simulink model "DiscreteDroneModelV2"  (R2024a)
settings: Solver=VariableStepAuto  StartTime=0.0  StopTime=20  RelTol=1e-3
PreLoadFcn:
  | run("StateSpace.m")
  | run("QuadcopterAttributes.m")
  | run("Motormixing.m")
  | run("reduced_state_space.m")
  | run("LQI_reduced.m")
values from neighbouring files (symbols this model uses):
  A_r = [0 0 0 0 1 0 0 0 ... (first row only)    [reduced_state_space.m]
  B = [0 0 0 0 ... (first row only)    [StateSpace.m]
  B_r = [0 0 0 0 ... (first row only)    [reduced_state_space.m]
  C = [1 0 0 0 0 0 0 0 0 0 0 0 ... (first row only)    [StateSpace.m]
  C_r = ctrb(A,B)    [OptimalControlLQCalculations.m]    (also in reduced_state_space.m = [1 0 0 0 0 0 0 0)
  dis = 81.17 * 10^-3    (= 0.08117)    [Motormixing.m]
  drag_co = torque_Nm / no_rot^2    (= 9.75332775919e-12)    [QuadcopterAttributes.m]
  E = [1 0 0 0 0 0 0 0;]    [LQI_reduced.m]
  g = 9.81    [StateSpace.m]
  K_LQR_reduced = lqr(A_r, B_r, Q_reduced, R_reduced, 0)    [LQR_reduced.m]    (also in reduced_state_space.m)
  K_mm = inv(K_mm_FtoU)    [Motormixing.m]
  Ki_lqi = K_lqi(:,13:16)    [LQI.m]    (also in LQICalculations.m)
  Ki_lqi_reduced = K_lqi_reduced(:,9)    [LQI_reduced.m]
  KV_rating = 2800    [QuadcopterAttributes.m]
  Kx_lqi = K_lqi(:,1:12)    [LQI.m]    (also in LQICalculations.m)
  Kx_lqi_reduced = K_lqi_reduced(:,1:8)    [LQI_reduced.m]
  lift_co = thrust_N / no_rot^2    (= 5.88883004597e-10)    [QuadcopterAttributes.m]
  m = 0.5    [StateSpace.m]
  r = 0.25    [StateSpace.m]
  x0_r = [0;0;0;0;0;0;0;0;]    [reduced_state_space.m]
undefined symbols (not defined in the file or in its folder): A, battery_voltage, C_lqi, I_p, sigma
libraries: sim3dlib x2, uavsim3dlib x2, shared6dof x1
settings Model: Creator=Henrik  LastModifiedBy=felih

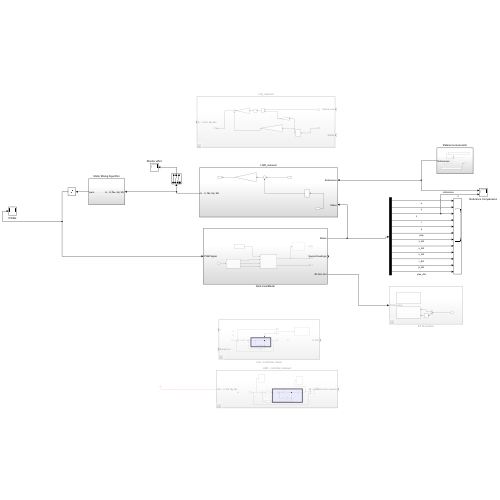
[thumbnail: Simulink's stored preview of the top-level diagram]
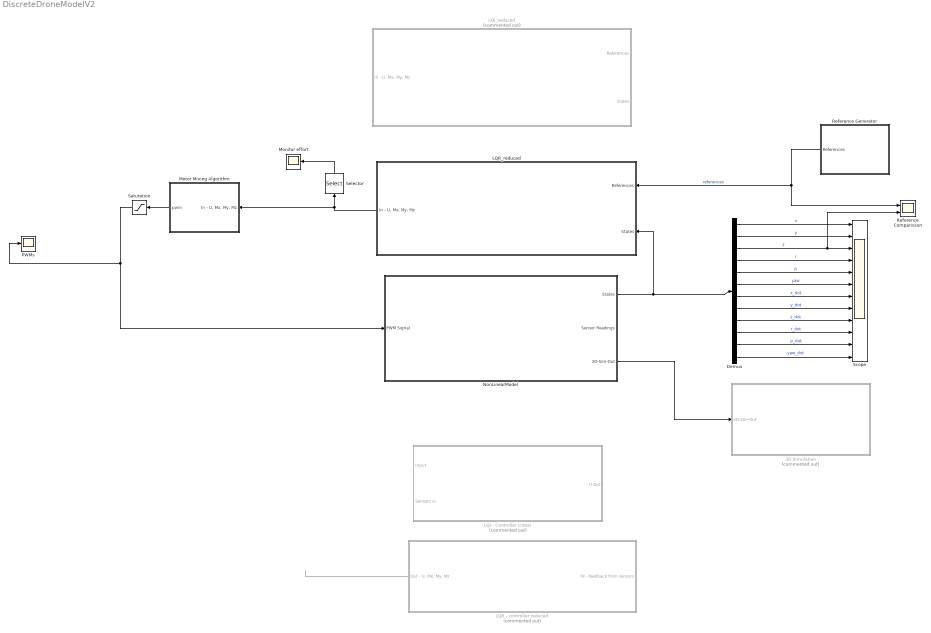
== system DiscreteDroneModelV2 ==
  3D Simulation : Subsystem  Commented=on
  Demux : Demux  Outputs=12
  LQI - Controller Linear : Subsystem  Commented=on
  LQI_reduced : Subsystem  Commented=on
  LQR - controller reduced : Subsystem  Commented=on
  LQR_reduced : Subsystem
  Monitor effort : Scope
  Motor Mixing Algorithm : Subsystem
  NonLinearModel : Subsystem
  PWMs : Scope
  Reference Comparisson : Scope  NumInputPorts=2
  Reference Generator : Subsystem
  Saturation : Saturate  UpperLimit=255  LowerLimit=0
  Scope : Scope  NumInputPorts=12
  Selector : Selector  InputPortWidth=4  IndexOptions=Index vector (dialog)  Indices=[1 2 3]  OutputSizes=1
  wires:
  LQR - controller reduced/1("Out - U, Mx, My, Mz") -> ?
  Demux/1 -> Scope/1  "x"
  Demux/2 -> Scope/2  "y"
  Demux/3 -> Reference Comparisson/2, Scope/3  "z"
  Demux/4 -> Scope/4  "r"
  Demux/5 -> Scope/5  "p"
  Demux/6 -> Scope/6  "yaw"
  Demux/7 -> Scope/7  "x_dot"
  Demux/8 -> Scope/8  "y_dot"
  Demux/9 -> Scope/9  "z_dot"
  Demux/10 -> Scope/10  "r_dot"
  Demux/11 -> Scope/11  "p_dot"
  Demux/12 -> Scope/12  "yaw_dot"
  NonLinearModel/1(States) -> LQR_reduced/2(States), Demux/1
  Motor Mixing Algorithm/1(pwm) -> Saturation/1
  Saturation/1 -> PWMs/1, NonLinearModel/1(PWM Signal)
  LQR_reduced/1("In - U, Mx, My, Mz") -> Selector/1, Motor Mixing Algorithm/1("In - U, Mx, My, Mz")
  Reference Generator/1(References) -> Reference Comparisson/1, LQR_reduced/1(References)  "references"
  Selector/1 -> Monitor effort/1
  NonLinearModel/3(3D-Sim-Out) -> 3D Simulation/1(3D-Sim-Out)

== system DiscreteDroneModelV2/3D Simulation ==
  3D-Sim-Out : Inport
  Demux : Demux  Outputs=2
  Flip : DSPFlip
  Simulation 3D Scene Configuration : sim3dlib/Simulation 3D Scene Configuration  Priority=0  ProjectFormat=Default Scenes  SceneDesc=US city block  ProjectName=C:\Program Files\MATLAB\R2024a\toolbox\shared\sim3d_projects\automotive_project_windows\UE\WindowsNoEditor\VehicleSimulation.exe  ScenePath=/Game/Maps/USCityBlock  EnableOpenDRIVE=off  vehTagList={'Scene Origin';'SimulinkVehicle1'}  vehTag=SimulinkVehicle1  FreeCameraInitialTranslation=[0, 0, 0]  FreeCameraDefaultInitialTranslation=[-6, 0, 2]  FreeCameraInitialRotation=[0, 0, 0]  FreeCameraDefaultInitialRotation=[0, -15, 0]  OpVisEn=off  Ts=1/60  EnableWindow=on  EnableRemoteAccess=off  EnableWeather=off  SunAzimuth=90  SunAltitude=40.0  EnableGeospatialSun=off  Latitude=0  Longitude=0  Date=2023-01-01  Time=10:30:00  GeoTimeZone=-5.0  SunDaylightSaving=off  wind=1  clouds=10  EnableVolumetricClouds=off  CloudCoverage=0  CloudAltitude=6  fog=30.0  rain=0  RaindropsEffect=off  SnowDensity=0  EnableGeospatial=off  UseTrueOrigin=off  OriginHeight=200  OriginLatitude=40.744652  OriginLongitude=-73.988864  MapStyle=Aerial  AdditionalAssetIDs=[]  UseAdvancedSunSky=off  SolarTime=11  TimeZone=-5  Day=21  Month=9  Year=2022  UseDaylightSavingTime=on  DSTStartDay=10  DSTStartMonth=3  DSTEndDay=3  DSTEndMonth=11  DSTSwitchHour=2  sensorTag=MainCamera1  sensorId=1  sensorName=MainCamera1  mountLoc=Origin  offsetFlag=off  tmountOffset=[0, 0, 0]  rmountOffset=[0, 0, 0]  HorizontalResolution=1280  VerticalResolution=720  HorizontalFOV=60  mountPoint=[0 0 0]  mountOrientation=[0 0 0]  aMode=4  ID=1  GeoTrigger=Inactive
      settings: LibrarySourceBlock=uavsim3dlib/Simulation 3D Scene Configuration
  Simulation 3D UAV Vehicle : uavsim3dlib/Simulation 3D UAV Vehicle  Priority=-1  Mesh=Quadrotor  MeshPath=/MathWorksUAVContent/UAVs/HexaRotorUAV/HexaRotor.HexaRotor  Color=Silver  ActorName=SimulinkVehicle1  UseGlobalFrame=off  InitialTranslation=[0 0 0]  InitialRotation=[0 0 0]  InitialTranslationGlobal=[0 0 0]  InitialGeoOrigin=[0 0 0]  InitialRotationGlobal=[0 0 0]  SampleTime=-1  ActorType=SimulinkVehicle  ID=1  aMode=4  ActorTag=SimulinkVehicle1
  wires:
  Demux/1 -> Simulation 3D UAV Vehicle/1
  Flip/1 -> Simulation 3D UAV Vehicle/2
  Demux/2 -> Flip/1
  3D-Sim-Out/1 -> Demux/1

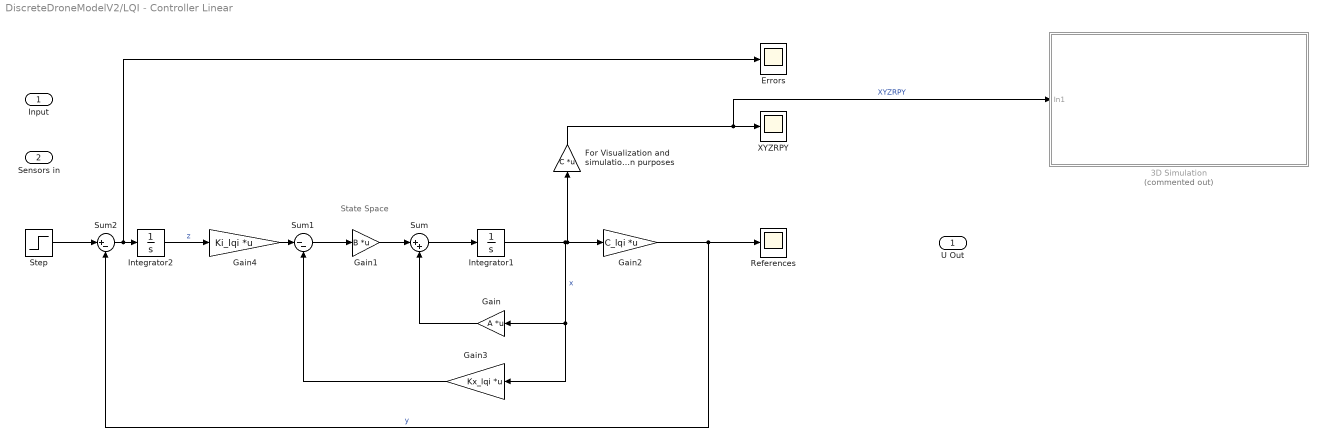
== system DiscreteDroneModelV2/LQI - Controller Linear ==
  note: State Space
  Input : Inport
  Sensors in : Inport  Port=2
  3D Simulation : Subsystem  Commented=on
  Errors : Scope
  For Visualization and simulation purposes : Gain  Gain=C  Multiplication=Matrix(K*u)
  Gain : Gain  Gain=A  Multiplication=Matrix(K*u)
  Gain1 : Gain  Gain=B  Multiplication=Matrix(K*u)
  Gain2 : Gain  Gain=C_lqi  Multiplication=Matrix(K*u)
  Gain3 : Gain  Gain=Kx_lqi  Multiplication=Matrix(K*u)
  Gain4 : Gain  Gain=Ki_lqi  Multiplication=Matrix(K*u)
  Integrator1 : Integrator
  Integrator2 : Integrator
  References : Scope
  Step : Step  Before=[0;0;0;0]  After=[20;-3;100;3]  SampleTime=0
  Sum : Sum  Inputs=|++
  Sum1 : Sum  Inputs=|--
  Sum2 : Sum  Inputs=|+-
  XYZRPY : Scope
  U Out : Outport
  wires:
  Gain/1 -> Sum/2
  Gain1/1 -> Sum/1
  Sum/1 -> Integrator1/1
  Integrator1/1 -> For Visualization and simulation purposes/1, Gain2/1, Gain3/1, Gain/1  "x"
  Gain2/1 -> References/1, Sum2/2  "y"
  Sum1/1 -> Gain1/1
  Gain3/1 -> Sum1/2
  Step/1 -> Sum2/1
  Sum2/1 -> Errors/1, Integrator2/1
  Integrator2/1 -> Gain4/1  "z"
  Gain4/1 -> Sum1/1
  For Visualization and simulation purposes/1 -> 3D Simulation/1(In1), XYZRPY/1  "XYZRPY"

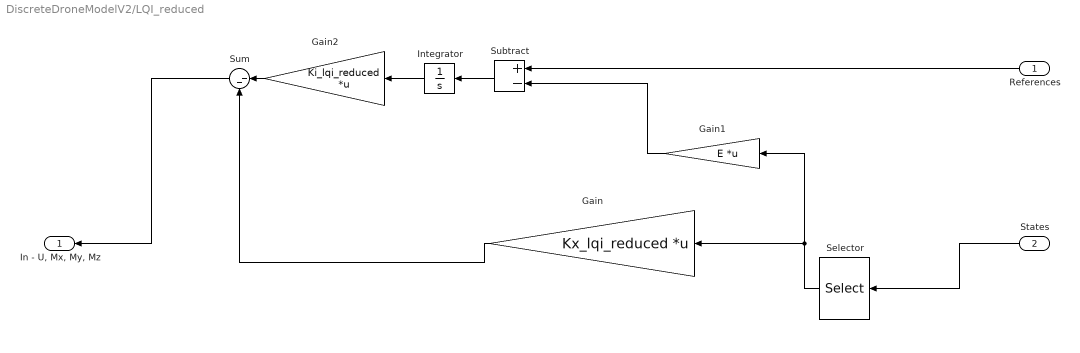
== system DiscreteDroneModelV2/LQI_reduced ==
  References : Inport
  States : Inport  Port=2
  Gain : Gain  Gain=Kx_lqi_reduced  Multiplication=Matrix(K*u)
  Gain1 : Gain  Gain=E  Multiplication=Matrix(K*u)
  Gain2 : Gain  Gain=Ki_lqi_reduced  Multiplication=Matrix(K*u)
  Integrator : Integrator
  Selector : Selector  InputPortWidth=12  IndexOptions=Index vector (dialog)  Indices=[3 4 5 6 9 10 11 12]  OutputSizes=1
  Subtract : Sum  Inputs=+-
  Sum : Sum  Inputs=|--
  "In - U, Mx, My, Mz" : Outport
  wires:
  Selector/1 -> Gain1/1, Gain/1
  Subtract/1 -> Integrator/1
  Gain1/1 -> Subtract/2
  Sum/1 -> "In - U, Mx, My, Mz"/1
  Gain/1 -> Sum/2
  Gain2/1 -> Sum/1
  Integrator/1 -> Gain2/1
  References/1 -> Subtract/1
  States/1 -> Selector/1

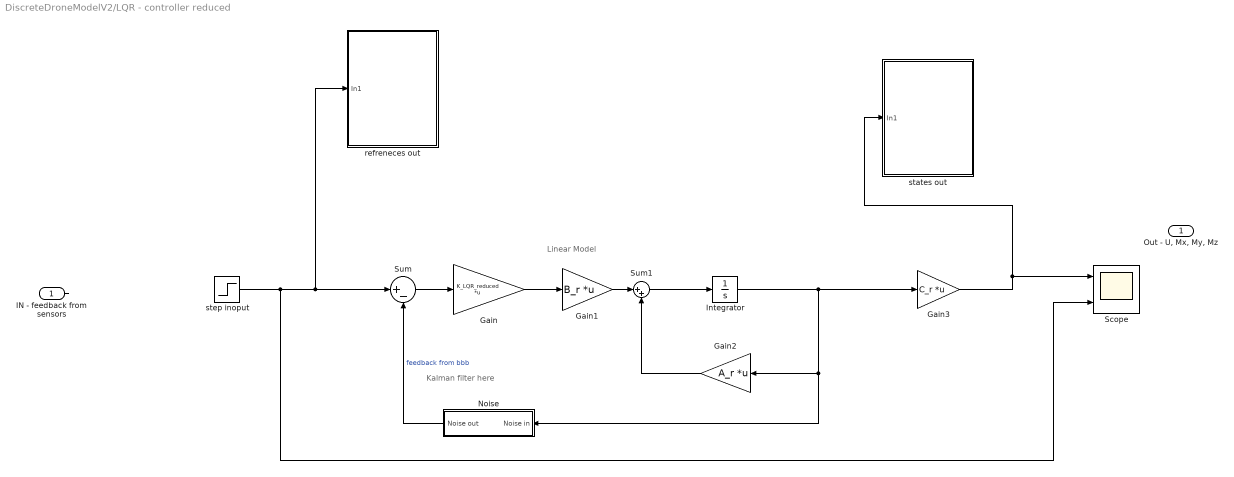
== system DiscreteDroneModelV2/LQR - controller reduced ==
  note: Linear Model
  note: Kalman filter here
  IN - feedback from sensors : Inport
  Gain : Gain  Gain=K_LQR_reduced  Multiplication=Matrix(K*u)
  Gain1 : Gain  Gain=B_r  Multiplication=Matrix(K*u)
  Gain2 : Gain  Gain=A_r  Multiplication=Matrix(K*u)
  Gain3 : Gain  Gain=C_r  Multiplication=Matrix(K*u)
  Integrator : Integrator  InitialCondition=x0_r
  Noise : Subsystem
  Scope : Scope  NumInputPorts=2
  Sum : Sum  Inputs=|+-
  Sum1 : Sum  Inputs=|++
  refreneces out : Subsystem
  states out : Subsystem
  step inoput : Step  Time=0  Before=zeros(8,1)  After=[0;1;0;0;0;0;0;0]  SampleTime=0
  "Out - U, Mx, My, Mz" : Outport
  wires:
  IN - feedback from sensors/1 -> ?
  Sum/1 -> Gain/1
  Gain/1 -> Gain1/1
  Gain1/1 -> Sum1/1
  Gain2/1 -> Sum1/2
  Sum1/1 -> Integrator/1
  Integrator/1 -> Gain2/1, Noise/1(Noise in), Gain3/1
  Gain3/1 -> states out/1(In1), Scope/1
  step inoput/1 -> Scope/2, refreneces out/1(In1), Sum/1
  Noise/1(Noise out) -> Sum/2  "feedback from bbb"

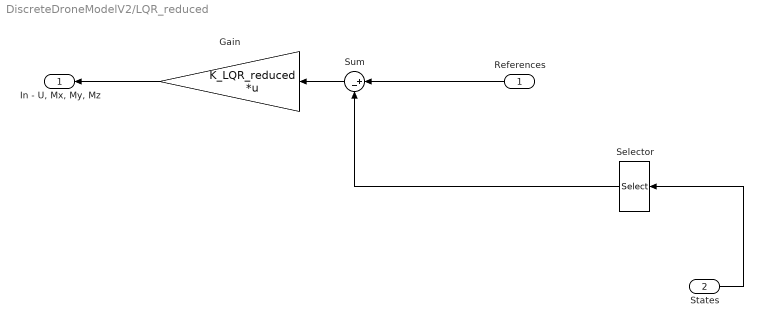
== system DiscreteDroneModelV2/LQR_reduced ==
  References : Inport
  States : Inport  Port=2
  Gain : Gain  Gain=K_LQR_reduced  Multiplication=Matrix(K*u)
  Selector : Selector  InputPortWidth=12  IndexOptions=Index vector (dialog)  Indices=[3 4 5 6 9 10 11 12]  OutputSizes=1
  Sum : Sum  Inputs=|+-
  "In - U, Mx, My, Mz" : Outport
  wires:
  Gain/1 -> "In - U, Mx, My, Mz"/1
  Selector/1 -> Sum/2
  Sum/1 -> Gain/1
  States/1 -> Selector/1
  References/1 -> Sum/1

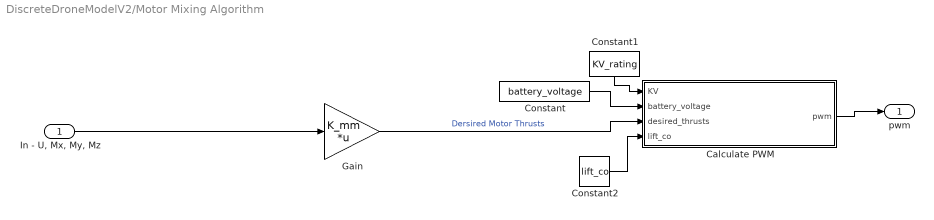
== system DiscreteDroneModelV2/Motor Mixing Algorithm ==
  "In - U, Mx, My, Mz" : Inport
  Calculate PWM : MATLAB Function  TreatAsAtomicUnit=on
  Constant : Constant  Value=battery_voltage
  Constant1 : Constant  Value=KV_rating
  Constant2 : Constant  Value=lift_co
  Gain : Gain  Gain=K_mm  Multiplication=Matrix(K*u)
  pwm : Outport
  wires:
  "In - U, Mx, My, Mz"/1 -> Gain/1
  Gain/1 -> Calculate PWM/3(desired_thrusts)  "Dersired Motor Thrusts"
  Constant/1 -> Calculate PWM/2(battery_voltage)
  Constant1/1 -> Calculate PWM/1(KV)
  Calculate PWM/1(pwm) -> pwm/1
  Constant2/1 -> Calculate PWM/4(lift_co)

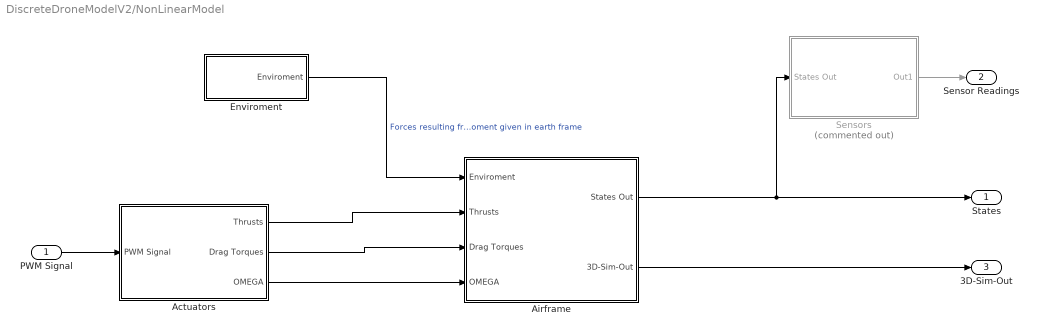
== system DiscreteDroneModelV2/NonLinearModel ==
  PWM Signal : Inport
  Actuators : Subsystem
  Airframe : Subsystem
  Enviroment : Subsystem
  Sensors : Subsystem  Commented=on
  States : Outport
  Sensor Readings : Outport  Port=2
  3D-Sim-Out : Outport  Port=3
  wires:
  PWM Signal/1 -> Actuators/1(PWM Signal)
  Airframe/1(States Out) -> Sensors/1(States Out), States/1
  Enviroment/1(Enviroment) -> Airframe/1(Enviroment)  "Forces resulting from enviroment given in earth frame"
  Actuators/1(Thrusts) -> Airframe/2(Thrusts)
  Airframe/2(3D-Sim-Out) -> 3D-Sim-Out/1
  Actuators/2(Drag Torques) -> Airframe/3(Drag Torques)
  Actuators/3(OMEGA) -> Airframe/4(OMEGA)
  Sensors/1(Out1) -> Sensor Readings/1

== system DiscreteDroneModelV2/Reference Generator ==
  Constant : Constant  Value=[0;0;0;0;0;0;0]
  Constant1 : Constant  Value=[0.35;0;0;0;0;0;0;0]
  Mux : Mux  Inputs=2
  Step : Step  Time=0  After=0.35  SampleTime=0
  References : Outport
  wires:
  Step/1 -> ?
  Constant/1 -> Mux/2
  Mux/1 -> ?
  Constant1/1 -> References/1

== system DiscreteDroneModelV2/LQI - Controller Linear/3D Simulation ==
  In1 : Inport
  Demux : Demux  Outputs=2
  Flip : DSPFlip
  Simulation 3D Scene Configuration : sim3dlib/Simulation 3D Scene Configuration  Priority=0  ProjectFormat=Default Scenes  SceneDesc=US city block  ProjectName=C:\Program Files\MATLAB\R2024a\toolbox\shared\sim3d_projects\automotive_project_windows\UE\WindowsNoEditor\VehicleSimulation.exe  ScenePath=/Game/Maps/USCityBlock  EnableOpenDRIVE=off  vehTagList={'Scene Origin';'SimulinkVehicle1'}  vehTag=SimulinkVehicle1  FreeCameraInitialTranslation=[0, 0, 0]  FreeCameraDefaultInitialTranslation=[-6, 0, 2]  FreeCameraInitialRotation=[0, 0, 0]  FreeCameraDefaultInitialRotation=[0, -15, 0]  OpVisEn=off  Ts=1/60  EnableWindow=on  EnableRemoteAccess=off  EnableWeather=off  SunAzimuth=90  SunAltitude=40.0  EnableGeospatialSun=off  Latitude=0  Longitude=0  Date=2023-01-01  Time=10:30:00  GeoTimeZone=-5.0  SunDaylightSaving=off  wind=1  clouds=10  EnableVolumetricClouds=off  CloudCoverage=0  CloudAltitude=6  fog=30.0  rain=0  RaindropsEffect=off  SnowDensity=0  EnableGeospatial=off  UseTrueOrigin=off  OriginHeight=200  OriginLatitude=40.744652  OriginLongitude=-73.988864  MapStyle=Aerial  AdditionalAssetIDs=[]  UseAdvancedSunSky=off  SolarTime=11  TimeZone=-5  Day=21  Month=9  Year=2022  UseDaylightSavingTime=on  DSTStartDay=10  DSTStartMonth=3  DSTEndDay=3  DSTEndMonth=11  DSTSwitchHour=2  sensorTag=MainCamera1  sensorId=1  sensorName=MainCamera1  mountLoc=Origin  offsetFlag=off  tmountOffset=[0, 0, 0]  rmountOffset=[0, 0, 0]  HorizontalResolution=1280  VerticalResolution=720  HorizontalFOV=60  mountPoint=[0 0 0]  mountOrientation=[0 0 0]  aMode=4  ID=1  GeoTrigger=Inactive
      settings: LibrarySourceBlock=uavsim3dlib/Simulation 3D Scene Configuration
  Simulation 3D UAV Vehicle : uavsim3dlib/Simulation 3D UAV Vehicle  Priority=-1  Mesh=Quadrotor  MeshPath=/MathWorksUAVContent/UAVs/HexaRotorUAV/HexaRotor.HexaRotor  Color=Silver  ActorName=SimulinkVehicle1  UseGlobalFrame=off  InitialTranslation=[0 0 0]  InitialRotation=[0 0 0]  InitialTranslationGlobal=[0 0 0]  InitialGeoOrigin=[0 0 0]  InitialRotationGlobal=[0 0 0]  SampleTime=-1  ActorType=SimulinkVehicle  ID=1  aMode=4  ActorTag=SimulinkVehicle1
  wires:
  Demux/1 -> Simulation 3D UAV Vehicle/1
  Flip/1 -> Simulation 3D UAV Vehicle/2
  Demux/2 -> Flip/1
  In1/1 -> Demux/1

== system DiscreteDroneModelV2/LQR - controller reduced/Noise ==
  Noise in : Inport
  Random Number12 : RandomNumber  Mean=0.1  Variance=0.1  SampleTime=0.001
  Sum2 : Sum  Inputs=|++
  Transfer Fcn12 : TransferFcn  Numerator=[50 0]  Denominator=[50 1]
  X noise1 : Gain  Gain=[0;1;0;0;0;0;0;0]  Multiplication=Matrix(K*u)
  Noise out : Outport
  wires:
  X noise1/1 -> Sum2/2
  Transfer Fcn12/1 -> X noise1/1
  Random Number12/1 -> Transfer Fcn12/1
  Noise in/1 -> Sum2/1
  Sum2/1 -> Noise out/1

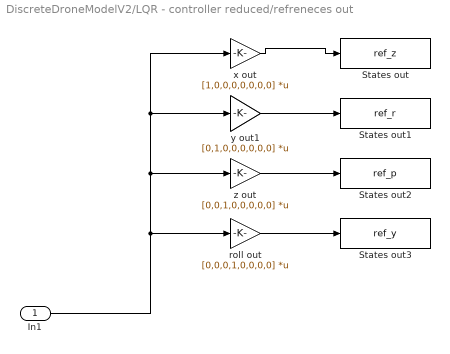
== system DiscreteDroneModelV2/LQR - controller reduced/refreneces out ==
  In1 : Inport
  States out : ToWorkspace  VariableName=ref_z  SaveFormat=Timeseries  SampleTime=-1
  States out1 : ToWorkspace  VariableName=ref_r  SaveFormat=Timeseries  SampleTime=-1
  States out2 : ToWorkspace  VariableName=ref_p  SaveFormat=Timeseries  SampleTime=-1
  States out3 : ToWorkspace  VariableName=ref_y  SaveFormat=Timeseries  SampleTime=-1
  roll out : Gain  Gain=[0,0,0,1,0,0,0,0]  Multiplication=Matrix(K*u)
  x out : Gain  Gain=[1,0,0,0,0,0,0,0]  Multiplication=Matrix(K*u)
  y out1 : Gain  Gain=[0,1,0,0,0,0,0,0]  Multiplication=Matrix(K*u)
  z out : Gain  Gain=[0,0,1,0,0,0,0,0]  Multiplication=Matrix(K*u)
  wires:
  z out/1 -> States out2/1
  In1/1 -> roll out/1, z out/1, y out1/1, x out/1
  y out1/1 -> States out1/1
  x out/1 -> States out/1
  roll out/1 -> States out3/1

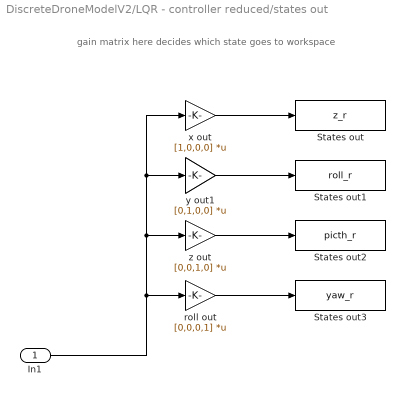
== system DiscreteDroneModelV2/LQR - controller reduced/states out ==
  note: gain matrix here decides which state goes to workspace
  In1 : Inport
  States out : ToWorkspace  VariableName=z_r  SaveFormat=Timeseries  SampleTime=-1
  States out1 : ToWorkspace  VariableName=roll_r  SaveFormat=Timeseries  SampleTime=-1
  States out2 : ToWorkspace  VariableName=picth_r  SaveFormat=Timeseries  SampleTime=-1
  States out3 : ToWorkspace  VariableName=yaw_r  SaveFormat=Timeseries  SampleTime=-1
  roll out : Gain  Gain=[0,0,0,1]  Multiplication=Matrix(K*u)
  x out : Gain  Gain=[1,0,0,0]  Multiplication=Matrix(K*u)
  y out1 : Gain  Gain=[0,1,0,0]  Multiplication=Matrix(K*u)
  z out : Gain  Gain=[0,0,1,0]  Multiplication=Matrix(K*u)
  wires:
  y out1/1 -> States out1/1
  In1/1 -> x out/1, y out1/1, z out/1, roll out/1
  roll out/1 -> States out3/1
  z out/1 -> States out2/1
  x out/1 -> States out/1

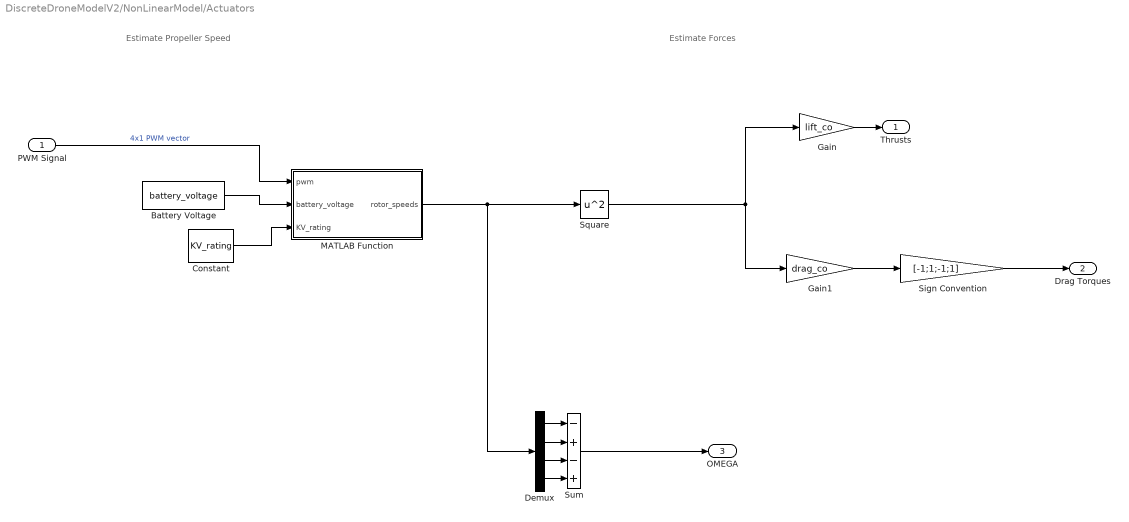
== system DiscreteDroneModelV2/NonLinearModel/Actuators ==
  note: Estimate Forces
  note: Estimate Propeller Speed
  PWM Signal : Inport
  Battery Voltage : Constant  Value=battery_voltage
  Constant : Constant  Value=KV_rating
  Demux : Demux
  Gain : Gain  Gain=lift_co
  Gain1 : Gain  Gain=drag_co
  MATLAB Function : MATLAB Function  TreatAsAtomicUnit=on
  Sign Convention : Gain  Gain=[-1;1;-1;1]
  Square : Math  Operator=square
  Sum : Sum  Inputs=-+-+
  Thrusts : Outport
  Drag Torques : Outport  Port=2
  OMEGA : Outport  Port=3
  wires:
  Constant/1 -> MATLAB Function/3(KV_rating)
  Battery Voltage/1 -> MATLAB Function/2(battery_voltage)
  PWM Signal/1 -> MATLAB Function/1(pwm)  "4x1 PWM vector"
  MATLAB Function/1(rotor_speeds) -> Square/1, Demux/1
  Gain/1 -> Thrusts/1
  Square/1 -> Gain/1, Gain1/1
  Gain1/1 -> Sign Convention/1
  Demux/1 -> Sum/1
  Demux/2 -> Sum/2
  Demux/3 -> Sum/3
  Demux/4 -> Sum/4
  Sum/1 -> OMEGA/1
  Sign Convention/1 -> Drag Torques/1

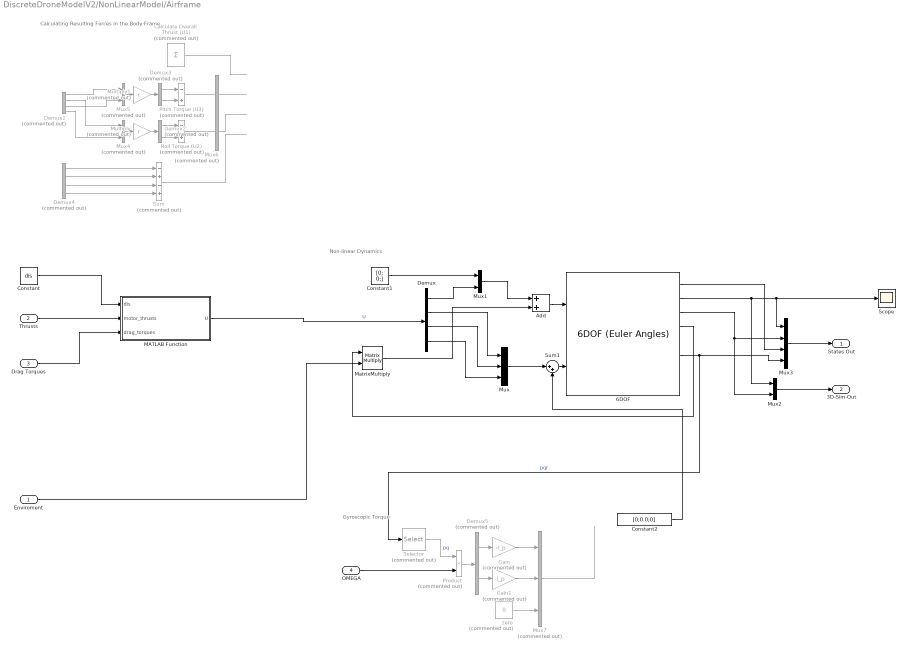
== system DiscreteDroneModelV2/NonLinearModel/Airframe ==
  note: Gyroscopic Torque
  note: Non-linear Dynamics
  note: Calculating Resulting Forces in the Body-Frame
  Enviroment : Inport
  Thrusts : Inport  Port=2
  Drag Torques : Inport  Port=3
  OMEGA : Inport  Port=4
  "6DOF " : shared6dof/6DOF (Euler Angles)  units=Metric (MKS)  mtype=Fixed  rep=Quaternion  xme_0=[0 0 0]  Vm_0=[0 0 0]  eul_0=[0 0 0]  pm_0=[0 0 0]  mass_0=m  mass_e=0.5  mass_f=2.0  inertia=Inertia_Mat  inertia_e=eye(3)  inertia_f=2*eye(3)  k_quat=1.0  vre_flag=on  abi_flag=off  aMode=0  xme_statename=''  Vm_statename=''  eul_statename=''  quat_statename=''  pm_statename=''  mass_statename=''
      settings: LibrarySourceBlock=aerolib6dof2/6DOF (Quaternion)
  Add : Sum
  "Calculate Overall Thrust (U1) " : Sum  Commented=on  Inputs=+
  Constant : Constant  Value=dis
  Constant1 : Constant  Value=[0; 0;]
  Constant2 : Constant  Value=[0;0.0;0]
  Demux : Demux
  Demux1 : Demux  Commented=on
  Demux2 : Demux  Commented=on  Outputs=2
  Demux3 : Demux  Commented=on  Outputs=2
  Demux4 : Demux  Commented=on
  Demux5 : Demux  Commented=on  Outputs=2
  Gain : Gain  Commented=on  Gain=-I_p
  Gain1 : Gain  Commented=on  Gain=I_p
  MATLAB Function : MATLAB Function  TreatAsAtomicUnit=on
  MatrixMultiply : Product  Multiplication=Matrix(*)
  Multiply : Gain  Commented=on  Gain=r
  Multiply1 : Gain  Commented=on  Gain=r
  Mux : Mux  Inputs=3
  Mux1 : Mux  Inputs=2
  Mux2 : Mux  Inputs=2
  Mux3 : Mux
  Mux4 : Mux  Commented=on  Inputs=2
  Mux5 : Mux  Commented=on  Inputs=2
  Mux6 : Mux  Commented=on
  Mux7 : Mux  Commented=on  Inputs=3
  Pitch Torque (U3) : Sum  Commented=on  Inputs=-+
  Product : Product  Commented=on
  Roll Torque (U2) : Sum  Commented=on  Inputs=-+
  Scope : Scope
  Selector : Selector  Commented=on  InputPortWidth=3  IndexOptions=Index vector (dialog)  Indices=[1 2]  OutputSizes=1
  Sum : Sum  Commented=on  Inputs=-+-+
  Sum1 : Sum  Inputs=|++
  zero : Constant  Commented=on  Value=0
  States Out : Outport
  3D-Sim-Out : Outport  Port=2
  wires:
  Demux/2 -> Mux/1
  Demux/3 -> Mux/2
  Demux/4 -> Mux/3
  Enviroment/1 -> MatrixMultiply/2
  "6DOF "/4 -> MatrixMultiply/1
  Add/1 -> "6DOF "/1
  MatrixMultiply/1 -> Add/2
  "6DOF "/2 -> Mux2/1, Mux3/1, Scope/1
  Demux/1 -> Mux1/2
  Constant1/1 -> Mux1/1
  Mux1/1 -> Add/1
  Mux2/1 -> 3D-Sim-Out/1
  "6DOF "/3 -> Mux3/2, Mux2/2
  "6DOF "/1 -> Mux3/3
  "6DOF "/6 -> Mux3/4, Selector/1  "pqr"
  Mux3/1 -> States Out/1
  MATLAB Function/1(U) -> Demux/1  "U"
  OMEGA/1 -> Product/2
  Selector/1 -> Product/1  "pq"
  Product/1 -> Demux5/1
  Demux5/1 -> Gain/1
  Demux5/2 -> Gain1/1
  Gain/1 -> Mux7/1
  Gain1/1 -> Mux7/2
  zero/1 -> Mux7/3
  Mux/1 -> Sum1/1
  Mux7/1 -> ?
  Sum1/1 -> "6DOF "/2
  Demux1/2 -> Mux4/1
  Demux4/3 -> Sum/3
  Demux2/1 -> Roll Torque (U2)/1
  Sum/1 -> ?
  Demux1/4 -> Mux4/2
  Multiply/1 -> Demux2/1
  Demux4/2 -> Sum/2
  Demux4/4 -> Sum/4
  Demux1/1 -> Mux5/1
  Demux3/1 -> Pitch Torque (U3)/1
  "Calculate Overall Thrust (U1) "/1 -> ?
  Demux4/1 -> Sum/1
  Roll Torque (U2)/1 -> ?
  ? -> "Calculate Overall Thrust (U1) "/1, Demux1/1
  Mux5/1 -> Multiply1/1
  Pitch Torque (U3)/1 -> ?
  Demux3/2 -> Pitch Torque (U3)/2
  Mux4/1 -> Multiply/1
  Demux1/3 -> Mux5/2
  Demux2/2 -> Roll Torque (U2)/2
  Multiply1/1 -> Demux3/1
  ? -> Demux4/1
  Constant/1 -> MATLAB Function/1(dis)
  Thrusts/1 -> MATLAB Function/2(motor_thrusts)
  Drag Torques/1 -> MATLAB Function/3(drag_torques)
  Constant2/1 -> Sum1/2

== system DiscreteDroneModelV2/NonLinearModel/Enviroment ==
  Gravity : Constant  Value=[0; 0; -m*g]
  Enviroment : Outport
  wires:
  Gravity/1 -> Enviroment/1  "Resulting Forces in the earth frame"

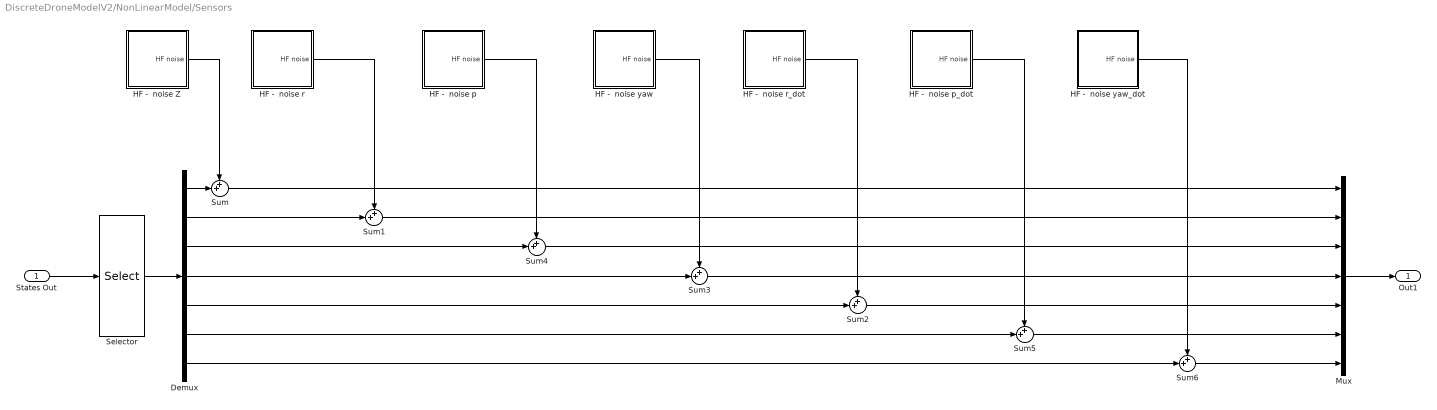
== system DiscreteDroneModelV2/NonLinearModel/Sensors ==
  States Out : Inport
  Demux : Demux  Outputs=7
  HF -  noise Z : Subsystem
  HF -  noise p : Subsystem
  HF -  noise p_dot : Subsystem
  HF -  noise r : Subsystem
  HF -  noise r_dot : Subsystem
  HF -  noise yaw : Subsystem
  HF -  noise yaw_dot : Subsystem
  Mux : Mux  Inputs=7
  Selector : Selector  InputPortWidth=12  IndexOptions=Index vector (dialog)  Indices=[3 4 5 6 10 11 12]  OutputSizes=1
  Sum{,1..6} (7 alike) : Sum  Inputs=++|
  Out1 : Outport
  wires:
  HF -  noise r/1(HF noise) -> Sum1/1
  HF -  noise p/1(HF noise) -> Sum4/1
  HF -  noise Z/1(HF noise) -> Sum/1
  HF -  noise yaw_dot/1(HF noise) -> Sum6/1
  HF -  noise yaw/1(HF noise) -> Sum3/1
  HF -  noise r_dot/1(HF noise) -> Sum2/1
  HF -  noise p_dot/1(HF noise) -> Sum5/1
  States Out/1 -> Selector/1
  Selector/1 -> Demux/1
  Demux/1 -> Sum/2
  Demux/2 -> Sum1/2
  Demux/3 -> Sum4/2
  Demux/4 -> Sum3/2
  Demux/5 -> Sum2/2
  Demux/6 -> Sum5/2
  Demux/7 -> Sum6/2
  Sum6/1 -> Mux/7
  Sum5/1 -> Mux/6
  Sum2/1 -> Mux/5
  Sum3/1 -> Mux/4
  Sum4/1 -> Mux/3
  Sum1/1 -> Mux/2
  Sum/1 -> Mux/1
  Mux/1 -> Out1/1

== system DiscreteDroneModelV2/NonLinearModel/Sensors/HF -  noise Z ==
  High pass filter : TransferFcn  Numerator=[50 0]  Denominator=[50 1]
  Noise : RandomNumber  Variance=sigma^2  SampleTime=0.01
  HF noise : Outport
  wires:
  Noise/1 -> High pass filter/1
  High pass filter/1 -> HF noise/1

== system DiscreteDroneModelV2/NonLinearModel/Sensors/HF -  noise p ==
  High pass filter : TransferFcn  Numerator=[50 0]  Denominator=[50 1]
  Noise : RandomNumber  Variance=sigma^2  SampleTime=0.01
  HF noise : Outport
  wires:
  Noise/1 -> High pass filter/1
  High pass filter/1 -> HF noise/1

== system DiscreteDroneModelV2/NonLinearModel/Sensors/HF -  noise p_dot ==
  High pass filter : TransferFcn  Numerator=[50 0]  Denominator=[50 1]
  Noise : RandomNumber  Variance=sigma^2  SampleTime=0.01
  HF noise : Outport
  wires:
  Noise/1 -> High pass filter/1
  High pass filter/1 -> HF noise/1

== system DiscreteDroneModelV2/NonLinearModel/Sensors/HF -  noise r ==
  High pass filter : TransferFcn  Numerator=[50 0]  Denominator=[50 1]
  Noise : RandomNumber  Variance=sigma^2  SampleTime=0.01
  HF noise : Outport
  wires:
  Noise/1 -> High pass filter/1
  High pass filter/1 -> HF noise/1

== system DiscreteDroneModelV2/NonLinearModel/Sensors/HF -  noise r_dot ==
  High pass filter : TransferFcn  Numerator=[50 0]  Denominator=[50 1]
  Noise : RandomNumber  Variance=sigma^2  SampleTime=0.01
  HF noise : Outport
  wires:
  Noise/1 -> High pass filter/1
  High pass filter/1 -> HF noise/1

== system DiscreteDroneModelV2/NonLinearModel/Sensors/HF -  noise yaw ==
  High pass filter : TransferFcn  Numerator=[50 0]  Denominator=[50 1]
  Noise : RandomNumber  Variance=sigma^2  SampleTime=0.01
  HF noise : Outport
  wires:
  Noise/1 -> High pass filter/1
  High pass filter/1 -> HF noise/1

== system DiscreteDroneModelV2/NonLinearModel/Sensors/HF -  noise yaw_dot ==
  High pass filter : TransferFcn  Numerator=[50 0]  Denominator=[50 1]
  Noise : RandomNumber  Variance=sigma^2  SampleTime=0.01
  HF noise : Outport
  wires:
  Noise/1 -> High pass filter/1
  High pass filter/1 -> HF noise/1

== matlab function DiscreteDroneModelV2/NonLinearModel/Airframe/MATLAB Function ==
  data: dis input; motor_thrusts input; U output; drag_torques input
function U = calc_U(dis, motor_thrusts, drag_torques)

    U = zeros(4,1); % Init U

    U(1,1) = sum(motor_thrusts); % Overall Thrust
    U(2,1) = dis * (motor_thrusts(1,1) + motor_thrusts(2,1) - (motor_thrusts(3,1) + motor_thrusts(4,1))); % Mx
    U(3,1) = dis * (motor_thrusts(2,1) + motor_thrusts(3,1) - (motor_thrusts(1,1) + motor_thrusts(4,1))); % My
    U(4,1) = sum(drag_torques); % Mz

== matlab function DiscreteDroneModelV2/NonLinearModel/Actuators/MATLAB Function ==
  data: pwm input; rotor_speeds output; battery_voltage input; KV_rating input
function rotor_speeds = fcn(pwm, battery_voltage, KV_rating)
    
    rotor_speeds = zeros(4,1); % Initialize rotor_speeds
    
    for i = 1:1:4
    
        duty_cycle = pwm(i,1)/255;
        rotor_speeds(i,1) = duty_cycle * battery_voltage * KV_rating;
    
    end

end

== matlab function DiscreteDroneModelV2/Motor Mixing Algorithm/Calculate PWM ==
  data: KV input; battery_voltage input; desired_thrusts input; pwm output; lift_co input
function pwm = calc_PWM(KV, battery_voltage, desired_thrusts, lift_co)

    pwm = zeros(4,1);
    req_rotorspeed = zeros (4,1);
    max_possible_rot_speed = battery_voltage * KV;

    for i = 1:1:4
        if desired_thrusts(i,1) > 0
            req_rotorspeed(i,1) = sqrt(desired_thrusts(i,1)/lift_co); % Estimate required rotor speeds
        else
            req_rotorspeed(i,1) = 0;
        end
        dutycycle = req_rotorspeed(i,1) / max_possible_rot_speed;
        pwm(i,1) = dutycycle * 255;
        
    end
